simulink model "DampedVibr"  (Simulink 10.2)
settings: Solver=VariableStepDiscrete  StartTime=0.0  StopTime=300.0  MaxStep=0.005  RelTol=1e-3
values from neighbouring files (symbols this model uses):
  F = 0.05    [DVibr.m]    (also in DampedVibr_In.m; Load_data2.m = 0.25)
  T = 50    [DVibr.m]    (also in DampedVibr_In.m; Load_data2.m = 80)
settings Model: Creator=Ranci  LastModifiedBy=Ranci
settings DataIOCC: SignalLoggingSaveFormat=Dataset  ReturnWorkspaceOutputs=on
settings OptimizationCC: LifeSpan=auto
settings DebuggingCC: UnderspecifiedInitializationDetection=Simplified  MergeDetectMultiDrivingBlocksExec=error  FcnCallInpInsideContextMsg=error  SFUnexpectedBacktrackingDiag=error  SFNoUnconditionalDefaultTransitionDiag=error  SFExecutionAtInitializationDiag=warning  ArithmeticOperatorsInVariantConditions=error
settings HardwareCC: ProdBitPerPointer=64  ProdBitPerSizeT=64  ProdBitPerPtrDiffT=64  ProdLargestAtomicFloat=Float  ProdIntDivRoundTo=Zero  ProdEndianess=LittleEndian  ProdWordSize=64  ProdHWDeviceType=Intel->x86-64 (Windows64)
settings ModelReferenceCC: PropagateSignalLabelsOutOfModel=on
settings SFSimCC: SimUseLocalCustomCode=on  CustomCodeUndefinedFunction=FilterOut
settings RTWCC: RTWUseLocalCustomCode=on
settings CodeAppCC: StateflowObjectComments=off
settings GRTTargetCC: TargetLangStandard=C99 (ISO)  CombineOutputUpdateFcns=on  GRTInterface=off
settings ConfigComp: CovMetricSettings=dwe  CovSaveCumulativeToWorkspaceVar=off  CovSaveSingleToWorkspaceVar=off  CovExternalEMLEnable=on

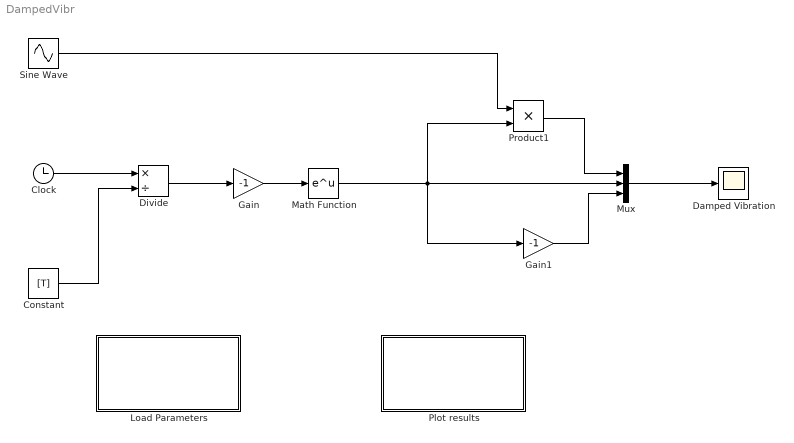
== system DampedVibr ==
  Clock : Clock
  Constant : Constant  Value=[T]
  Damped Vibration : Scope
  Divide : Product  Inputs=*/
  Gain : Gain  Gain=-1
  Gain1 : Gain  Gain=-1
  Load Parameters : Subsystem
      settings: OpenFcn=DampedVibr_In
      mask Display: disp('Press here\n to load parameters')
  Math Function : Math  SaturateOnIntegerOverflow=on
  Mux : Mux  Inputs=3
  Plot results : Subsystem
      settings: OpenFcn=DampedVibr_Out
      mask Display: disp('Press here\n to plot results')
  Product1 : Product
  Sine Wave : Sin  Frequency=2*pi*[F]  Phase=pi/2  SampleTime=0
  wires:
  Clock/1 -> Divide/1
  Constant/1 -> Divide/2
  Divide/1 -> Gain/1
  Gain/1 -> Math Function/1
  Sine Wave/1 -> Product1/1
  Product1/1 -> Mux/1
  Gain1/1 -> Mux/3
  Mux/1 -> Damped Vibration/1
  Math Function/1 -> Gain1/1, Product1/2, Mux/2

== system DampedVibr/Load Parameters ==

== system DampedVibr/Plot results ==
